simulink model "sim_mdlSensor_measData_16b"  (R2016b)
settings: Solver=ode4  StartTime=0.0  StopTime=10.0  FixedStep=0.0001  RelTol=1e-3
undefined symbols (not defined in the file or in its folder): Acc_uDot_mPerScnd2, Acc_vDot_mPerScnd2, Acc_wDot_mPerScnd2, AgVel_p_radPerScnd, AgVel_q_radPerScnd, AgVel_r_radPerScnd
settings Model: Creator=Nu  LastModifiedBy=Nu

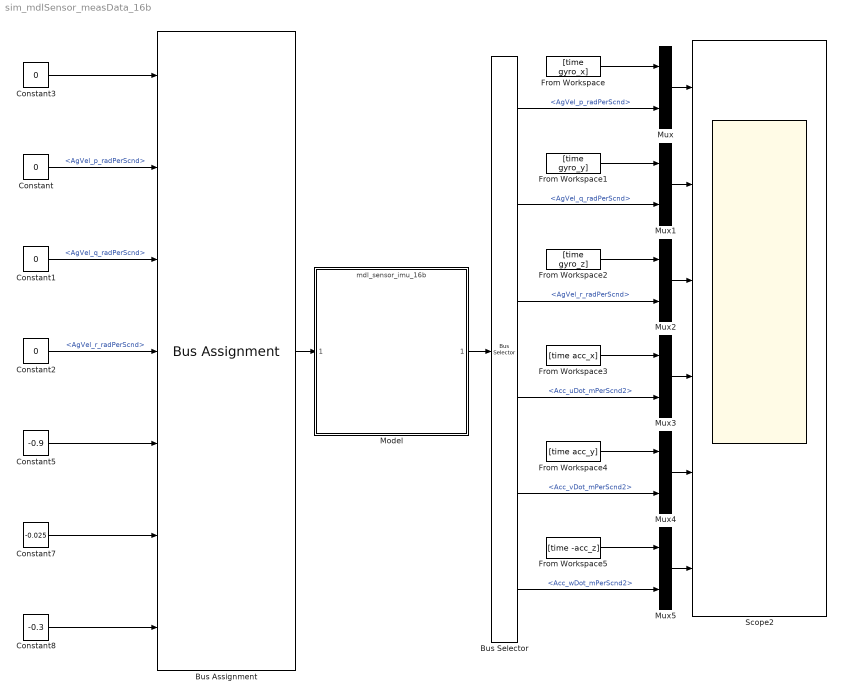
== system sim_mdlSensor_measData_16b ==
  Bus Assignment : BusAssignment  AssignedSignals=AgVel_p_radPerScnd,AgVel_q_radPerScnd,AgVel_r_radPerScnd,Acc_uDot_mPerScnd2,Acc_vDot_mPerScnd2,Acc_wDot_mPerScnd2
  Bus Selector : BusSelector  OutputSignals=AgVel_p_radPerScnd,AgVel_q_radPerScnd,AgVel_r_radPerScnd,Acc_uDot_mPerScnd2,Acc_vDot_mPerScnd2,Acc_wDot_mPerScnd2
  Constant : Constant  Value=0
  Constant1 : Constant  Value=0
  Constant2 : Constant  Value=0
  Constant3 : Constant  Value=0  OutDataTypeStr=Bus: mdl_statesExt
  Constant5 : Constant  Value=-0.9
  Constant7 : Constant  Value=-0.025
  Constant8 : Constant  Value=-0.3
  From Workspace : FromWorkspace  VariableName=[time gyro_x]  SampleTime=0
  From Workspace1 : FromWorkspace  VariableName=[time gyro_y]  SampleTime=0
  From Workspace2 : FromWorkspace  VariableName=[time gyro_z]  SampleTime=0
  From Workspace3 : FromWorkspace  VariableName=[time acc_x]  SampleTime=0
  From Workspace4 : FromWorkspace  VariableName=[time acc_y]  SampleTime=0
  From Workspace5 : FromWorkspace  VariableName=[time -acc_z]  SampleTime=0
  Model : ModelReference  ModelNameDialog=mdl_sensor_imu_16b.slx  SimulationMode=Normal  ModelReferenceVersion=1.231
  Mux{,1..5} (6 alike) : Mux  Inputs=2
  Scope2 : Scope  NumInputPorts=6
  wires:
  From Workspace1/1 -> Mux1/1
  Constant3/1 -> Bus Assignment/1
  Bus Assignment/1 -> Model/1
  Model/1 -> Bus Selector/1
  Constant/1 -> Bus Assignment/2  "<AgVel_p_radPerScnd>"
  Constant1/1 -> Bus Assignment/3  "<AgVel_q_radPerScnd>"
  Constant2/1 -> Bus Assignment/4  "<AgVel_r_radPerScnd>"
  Constant5/1 -> Bus Assignment/5
  Constant7/1 -> Bus Assignment/6
  Constant8/1 -> Bus Assignment/7
  Mux/1 -> Scope2/1
  Mux1/1 -> Scope2/2
  Mux2/1 -> Scope2/3
  Mux3/1 -> Scope2/4
  Mux4/1 -> Scope2/5
  Mux5/1 -> Scope2/6
  Bus Selector/1 -> Mux/2  "<AgVel_p_radPerScnd>"
  From Workspace/1 -> Mux/1
  Bus Selector/2 -> Mux1/2  "<AgVel_q_radPerScnd>"
  From Workspace2/1 -> Mux2/1
  Bus Selector/3 -> Mux2/2  "<AgVel_r_radPerScnd>"
  From Workspace3/1 -> Mux3/1
  Bus Selector/4 -> Mux3/2  "<Acc_uDot_mPerScnd2>"
  From Workspace4/1 -> Mux4/1
  From Workspace5/1 -> Mux5/1
  Bus Selector/6 -> Mux5/2  "<Acc_wDot_mPerScnd2>"
  Bus Selector/5 -> Mux4/2  "<Acc_vDot_mPerScnd2>"
